simulink model "Parallel_Inverter_Functional1"  (R2021a)
settings: Solver=ode23tb  StartTime=0.0  StopTime=2  RelTol=1e-3
InitFcn:
  | fsw=10e3;
  | Ts=50e-6;
  | Vodref=400*sqrt(2/3);
  | Vdc= 700;
  | w0=2*pi*50;
  | Vdref=400*sqrt(2/3);
  | Lf=3.5e-3;
  | Rf=0.1;
  | Cf=50e-6;
  | Lc1=0.3e-3;
  | Rc1=0.01;
  | Lc2=0.8e-3;
  | Rc2=0.05;
  | 
  | 
  | Tci=4/(2*pi*fsw);
  | wci=1/Tci;
  | Kpc=Lf*wci;
  | Kic=Rf*wci;
  | 
  | pm=50;
  | wcv=1/Tci*(1-sind(pm))/(1+sind(pm));
  | wgc=sqrt(wcv*wci);
  | Kpv=Cf*wgc;
  | Kiv=Kpv*wcv;
  | PLoad = 3000*0.8;
  | QLoad = 3000*0.6;
  | 
  | m1=5e-5;
  | n1=3e-4;
  | m2=2e-5;
  | n2=1e-4;
libraries: spsThreePhaseSeriesRLCBranchLib x6, spsabctodq0Lib x6, spsThreePhaseVIMeasurementLib x5, spsDCVoltageSourceLib x2, spsPWMGenerator2LevelLib x2, spsUniversalBridgeLib x2, spsGroundLib x2, spsdq0toabcLib x2, spsThreePhaseSeriesRLCLoadLib x2, spsThreePhaseBreakerLib x1, spspowerguiLib x1
settings Model: SimulationMode=accelerator  Creator=adarshadhungel1  LastModifiedBy=Electrical
settings SolverCC: AlgebraicLoopSolver=TrustRegion
settings DataIOCC: LoggingToFile=on
settings DebuggingCC: SFMachineParentedDataDiag=warning  ArithmeticOperatorsInVariantConditions=warning
settings SFSimCC: SimUseLocalCustomCode=off  CustomCodeUndefinedFunction=UseInterfaceOnly
settings RTWCC: RTWUseLocalCustomCode=off

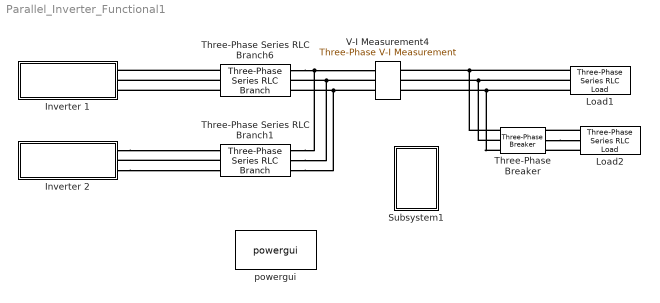
== system Parallel_Inverter_Functional1 ==
  Inverter 1 : Subsystem
  Inverter 2 : Subsystem
  Load1 : spsThreePhaseSeriesRLCLoadLib/Three-Phase Series RLC Load  LConnTagsString=A|B|C  Configuration=Y (grounded)  NominalVoltage=400  Vabc=[1e3 1e3 1e3]  Vabcp=[1e3 1e3 1e3]  NominalFrequency=50  UnbalancedPower=off  ActivePower=PLoad  InductivePower=QLoad  CapacitivePower=0  Pabc=[10e3 9e3 11e3]  QLabc=[100 90 110]  QCabc=[100 90 110]  Pabcp=[10e3 9e3 11e3]  QLabcp=[100 90 110]  QCabcp=[100 90 110]  Measurements=None  LoadType=constant Z
  Load2 : spsThreePhaseSeriesRLCLoadLib/Three-Phase Series RLC Load  LConnTagsString=A|B|C  Configuration=Y (grounded)  NominalVoltage=400  Vabc=[1e3 1e3 1e3]  Vabcp=[1e3 1e3 1e3]  NominalFrequency=50  UnbalancedPower=off  ActivePower=800  InductivePower=600  CapacitivePower=0  Pabc=[10e3 9e3 11e3]  QLabc=[100 90 110]  QCabc=[100 90 110]  Pabcp=[10e3 9e3 11e3]  QLabcp=[100 90 110]  QCabcp=[100 90 110]  Measurements=None  LoadType=constant Z
  Subsystem1 : Subsystem
  Three-Phase Series RLC Branch1 : spsThreePhaseSeriesRLCBranchLib/Three-Phase Series RLC Branch  LConnTagsString=A|B|C  RConnTagsString=A|B|C  BranchType=RL  Resistance=Rc2  Inductance=Lc2  Capacitance=1e-6  Measurements=None
  Three-Phase Series RLC Branch6 : spsThreePhaseSeriesRLCBranchLib/Three-Phase Series RLC Branch  LConnTagsString=A|B|C  RConnTagsString=A|B|C  BranchType=RL  Resistance=Rc1  Inductance=Lc1  Capacitance=1e-6  Measurements=None
  Three-Phase Breaker : spsThreePhaseBreakerLib/Three-Phase Breaker  InitialState=open  SwitchA=on  SwitchB=on  SwitchC=on  SwitchTimes="[1  2]"  External=off  BreakerResistance=0.01  SnubberResistance=1e6  SnubberCapacitance=inf  Measurements=None
  V-I Measurement4 : spsThreePhaseVIMeasurementLib/Three-Phase V-I Measurement  VoltageMeasurement=phase-to-ground  SetLabelV=on  LabelV=VLoad  Vpu=off  VpuLL=off  CurrentMeasurement=yes  SetLabelI=on  LabelI=ILoad  Ipu=off  Pbase=100e6  Vbase=500e3  OutputType=Complex  PhasorSimulation=off  PSBequivalent=0
  powergui : spspowerguiLib/powergui  Priority=1  SimulationMode=Discrete  SampleTime=Ts  frequency=60  Iterations=50  frequencyindice=0  Pbase=100e6  ErrMax=1e-4  UnitsV=kV  UnitsW=MW  buscounter=0  FunctionMessages=off  echomessages=off  EnableUseOfTLC=off  CurrentSourceSwitches=off  DisableSnubberDevices=off  DisableRonSwitches=off  DisableVfSwitches=off  DisplayEquations=off  AutomaticDiscreteSolvers=off  SolverType=Tustin/Backward Euler (TBE)  Interpol=off  ExternalGateDelay=off  methode=off  Ts=100  x0status=blocks  SPID=on  SwTol=0  HookPort=off  NonlinearTolerance=1e-4  nMaxIteration=100  ContinueOnMaxIteration=off  RestoreLinks=warning  ResistiveCurrentMeasurement=off  Frange=[0:2:500]  Ylog=off  Xlog=on  ShowGrid=off  save=off  variable=ZData  structure=VI1  ZoomFFT=off  StartTime=0  cycles=5  DisplayStyle=2  fundamental=50  FreqAxis=off  MaxFrequency=600  frequencyindicesteady=1  RmsSteady=1  display=off
  connections:
  Load1/LConn1 -- Three-Phase Breaker/LConn1 -- V-I Measurement4/RConn1
  Load1/LConn2 -- Three-Phase Breaker/LConn2 -- V-I Measurement4/RConn2
  Load1/LConn3 -- Three-Phase Breaker/LConn3 -- V-I Measurement4/RConn3
  Three-Phase Series RLC Branch6/RConn1 -- Three-Phase Series RLC Branch1/RConn1 -- V-I Measurement4/LConn1
  V-I Measurement4/LConn2 -- Three-Phase Series RLC Branch1/RConn2 -- Three-Phase Series RLC Branch6/RConn2
  V-I Measurement4/LConn3 -- Three-Phase Series RLC Branch1/RConn3 -- Three-Phase Series RLC Branch6/RConn3
  Three-Phase Series RLC Branch6/LConn1 -- Inverter 1/RConn1
  Three-Phase Series RLC Branch6/LConn2 -- Inverter 1/RConn2
  Three-Phase Series RLC Branch6/LConn3 -- Inverter 1/RConn3
  Inverter 2/RConn1 -- Three-Phase Series RLC Branch1/LConn1
  Three-Phase Series RLC Branch1/LConn2 -- Inverter 2/RConn2
  Inverter 2/RConn3 -- Three-Phase Series RLC Branch1/LConn3
  Load2/LConn1 -- Three-Phase Breaker/RConn1
  Three-Phase Breaker/RConn2 -- Load2/LConn2
  Load2/LConn3 -- Three-Phase Breaker/RConn3

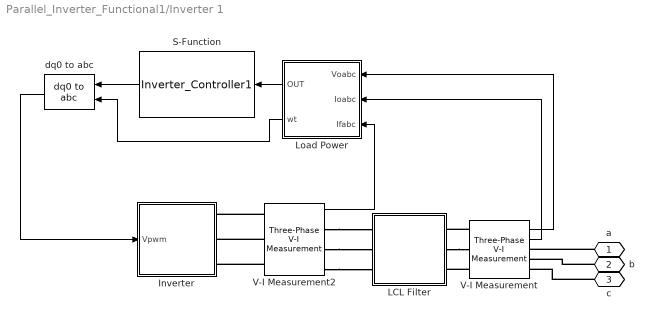
== system Parallel_Inverter_Functional1/Inverter 1 ==
  Inverter : Subsystem
  LCL Filter : Subsystem
  "Load Power " : Subsystem
  S-Function : S-Function  FunctionName=Inverter_Controller1  Parameters=Lf ,Cf  SFunctionDeploymentMode=off  EnableBusSupport=off
  V-I Measurement : spsThreePhaseVIMeasurementLib/Three-Phase V-I Measurement  VoltageMeasurement=phase-to-ground  SetLabelV=off  LabelV=Voabc  Vpu=off  VpuLL=off  CurrentMeasurement=yes  SetLabelI=off  LabelI=Ioabc  Ipu=off  Pbase=100e6  Vbase=500e3  OutputType=Complex  PhasorSimulation=off  PSBequivalent=0
  V-I Measurement2 : spsThreePhaseVIMeasurementLib/Three-Phase V-I Measurement  VoltageMeasurement=phase-to-ground  SetLabelV=on  LabelV=Viabc1  Vpu=off  VpuLL=off  CurrentMeasurement=yes  SetLabelI=off  LabelI=Ifabc  Ipu=off  Pbase=100e6  Vbase=500e3  OutputType=Complex  PhasorSimulation=off  PSBequivalent=0
  dq0 to abc : spsdq0toabcLib/dq0 to abc  Alignment=90 degrees behind phase A axis
  a : PMIOPort  Side=Right
  b : PMIOPort  Port=2  Side=Right
  c : PMIOPort  Port=3  Side=Right
  wires:
  "Load Power "/1(OUT) -> S-Function/1
  V-I Measurement/1 -> "Load Power "/1(Voabc)
  V-I Measurement/2 -> "Load Power "/2(Ioabc)
  V-I Measurement2/1 -> "Load Power "/3(Ifabc)
  S-Function/1 -> dq0 to abc/1
  "Load Power "/2(wt) -> dq0 to abc/2
  dq0 to abc/1 -> Inverter/1(Vpwm)
  connections:
  V-I Measurement2/LConn1 -- Inverter/RConn1
  V-I Measurement2/RConn1 -- LCL Filter/LConn1
  V-I Measurement/LConn3 -- LCL Filter/RConn3
  V-I Measurement2/LConn2 -- Inverter/RConn2
  V-I Measurement2/RConn2 -- LCL Filter/LConn2
  V-I Measurement2/LConn3 -- Inverter/RConn3
  V-I Measurement2/RConn3 -- LCL Filter/LConn3
  V-I Measurement/LConn1 -- LCL Filter/RConn1
  LCL Filter/RConn2 -- V-I Measurement/LConn2
  c/RConn1 -- V-I Measurement/RConn3
  b/RConn1 -- V-I Measurement/RConn2
  a/RConn1 -- V-I Measurement/RConn1

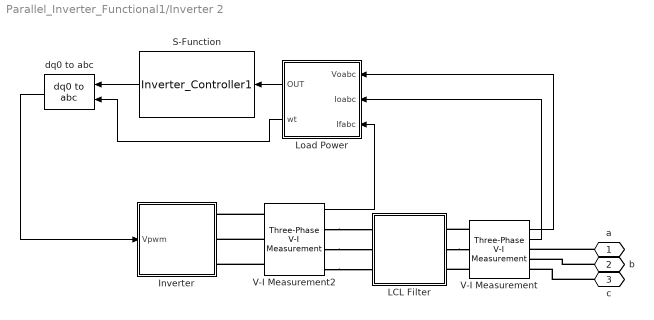
== system Parallel_Inverter_Functional1/Inverter 2 ==
  Inverter : Subsystem
  LCL Filter : Subsystem
  "Load Power " : Subsystem
  S-Function : S-Function  FunctionName=Inverter_Controller1  Parameters=Lf,Cf  SFunctionDeploymentMode=off  EnableBusSupport=off
  V-I Measurement : spsThreePhaseVIMeasurementLib/Three-Phase V-I Measurement  VoltageMeasurement=phase-to-ground  SetLabelV=off  LabelV=Voabc  Vpu=off  VpuLL=off  CurrentMeasurement=yes  SetLabelI=off  LabelI=Ioabc  Ipu=off  Pbase=100e6  Vbase=500e3  OutputType=Complex  PhasorSimulation=off  PSBequivalent=0
  V-I Measurement2 : spsThreePhaseVIMeasurementLib/Three-Phase V-I Measurement  VoltageMeasurement=phase-to-ground  SetLabelV=on  LabelV=Viabc  Vpu=off  VpuLL=off  CurrentMeasurement=yes  SetLabelI=off  LabelI=Ifabc  Ipu=off  Pbase=100e6  Vbase=500e3  OutputType=Complex  PhasorSimulation=off  PSBequivalent=0
  dq0 to abc : spsdq0toabcLib/dq0 to abc  Alignment=90 degrees behind phase A axis
  a : PMIOPort  Side=Right
  b : PMIOPort  Port=2  Side=Right
  c : PMIOPort  Port=3  Side=Right
  wires:
  dq0 to abc/1 -> Inverter/1(Vpwm)
  "Load Power "/2(wt) -> dq0 to abc/2
  S-Function/1 -> dq0 to abc/1
  V-I Measurement2/1 -> "Load Power "/3(Ifabc)
  V-I Measurement/2 -> "Load Power "/2(Ioabc)
  V-I Measurement/1 -> "Load Power "/1(Voabc)
  "Load Power "/1(OUT) -> S-Function/1
  connections:
  a/RConn1 -- V-I Measurement/RConn1
  b/RConn1 -- V-I Measurement/RConn2
  c/RConn1 -- V-I Measurement/RConn3
  LCL Filter/RConn2 -- V-I Measurement/LConn2
  V-I Measurement/LConn1 -- LCL Filter/RConn1
  V-I Measurement2/RConn3 -- LCL Filter/LConn3
  V-I Measurement2/LConn3 -- Inverter/RConn3
  V-I Measurement2/RConn2 -- LCL Filter/LConn2
  V-I Measurement2/LConn2 -- Inverter/RConn2
  V-I Measurement/LConn3 -- LCL Filter/RConn3
  V-I Measurement2/RConn1 -- LCL Filter/LConn1
  V-I Measurement2/LConn1 -- Inverter/RConn1

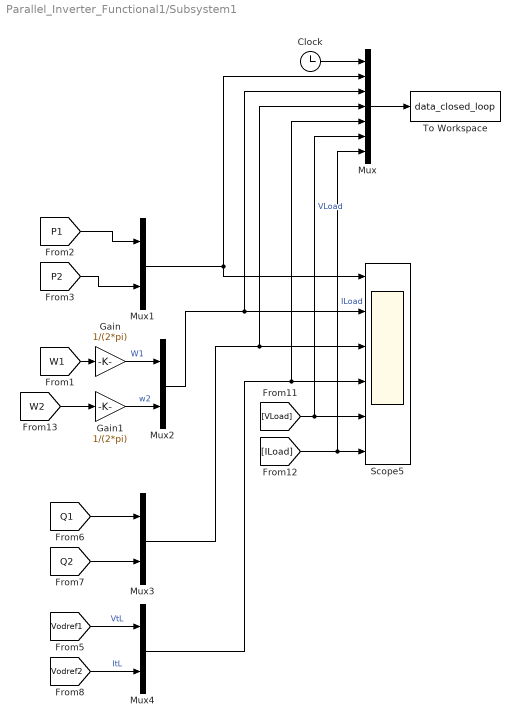
== system Parallel_Inverter_Functional1/Subsystem1 ==
  Clock : Clock
  Gain : Gain  Gain=1/(2*pi)
  Gain1 : Gain  Gain=1/(2*pi)
  Mux : Mux  Inputs=7
  Mux{1..4} (4 alike) : Mux  Inputs=2
  Scope5 : Scope  NumInputPorts=6
  To Workspace : ToWorkspace  VariableName=data_closed_loop  SampleTime=0.001
  wires:
  Mux3/1 -> Mux/4, Scope5/3
  Mux1/1 -> Scope5/1, Mux/2
  [Q1] -> Mux3/1
  [P1] -> Mux1/1
  Gain/1 -> Mux2/1  "W1"
  Mux4/1 -> Mux/5, Scope5/4
  [W2] -> Gain1/1
  [Vodref2] -> Mux4/2  "ItL"
  Mux2/1 -> Mux/3, Scope5/2
  Gain1/1 -> Mux2/2  "w2"
  [Q2] -> Mux3/2
  [VLoad] -> Mux/6, Scope5/5  "VLoad"
  [ILoad] -> Mux/7, Scope5/6  "ILoad"
  Clock/1 -> Mux/1
  [P2] -> Mux1/2
  Mux/1 -> To Workspace/1
  [W1] -> Gain/1
  [Vodref1] -> Mux4/1  "VtL"

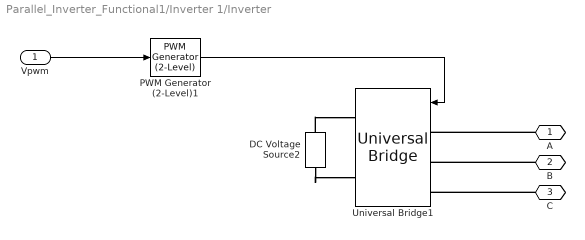
== system Parallel_Inverter_Functional1/Inverter 1/Inverter ==
  Vpwm : Inport
  DC Voltage Source2 : spsDCVoltageSourceLib/DC Voltage Source  Amplitude=Vdc  Measurements=None
  PWM Generator (2-Level)1 : spsPWMGenerator2LevelLib/PWM Generator (2-Level)  ModulatorType=Three-phase bridge (6 pulses)  ModulatorMode=Unsynchronized  Fc=fsw  Pc=0  nF=27  MinMax="[ -1  1 ]"  SamplingTechnique=Natural  ModulatingSignals=off  m=0.8  Freq=60  Phase=0  Ts=0  ShowCarrierOutport=off
  Universal Bridge1 : spsUniversalBridgeLib/Universal Bridge  Arms=3  SnubberResistance=1e5  SnubberCapacitance=inf  Device=IGBT / Diodes  Ron=1e-3  Lon=0  ForwardVoltages="[  0  0  ]"  ForwardVoltage=0  GTOparameters=[ 10e-6 , 20e-6 ]  IGBTparameters=[ 1e-6 , 2e-6 ]  Measurements=None  Measurements_2=None  converterType=Rectifier
  A : PMIOPort  Side=Right
  B : PMIOPort  Port=2  Side=Right
  C : PMIOPort  Port=3  Side=Right
  wires:
  PWM Generator (2-Level)1/1 -> Universal Bridge1/1
  Vpwm/1 -> PWM Generator (2-Level)1/1
  connections:
  A/RConn1 -- Universal Bridge1/LConn1
  C/RConn1 -- Universal Bridge1/LConn3
  DC Voltage Source2/LConn1 -- Universal Bridge1/RConn2
  DC Voltage Source2/RConn1 -- Universal Bridge1/RConn1
  B/RConn1 -- Universal Bridge1/LConn2

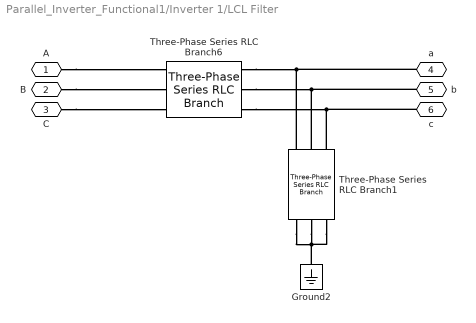
== system Parallel_Inverter_Functional1/Inverter 1/LCL Filter ==
  Ground2 : spsGroundLib/Ground  LConnTagsString=a
  Three-Phase Series RLC Branch1 : spsThreePhaseSeriesRLCBranchLib/Three-Phase Series RLC Branch  LConnTagsString=A|B|C  RConnTagsString=A|B|C  BranchType=C  Resistance=0.15  Inductance=3.5e-4  Capacitance=Cf  Measurements=None
  Three-Phase Series RLC Branch6 : spsThreePhaseSeriesRLCBranchLib/Three-Phase Series RLC Branch  LConnTagsString=A|B|C  RConnTagsString=A|B|C  BranchType=RL  Resistance=Rf  Inductance=Lf  Capacitance=1e-6  Measurements=None
  A : PMIOPort  Side=Left
  B : PMIOPort  Port=2  Side=Left
  C : PMIOPort  Port=3  Side=Left
  a : PMIOPort  Port=4  Side=Right
  b : PMIOPort  Port=5  Side=Right
  c : PMIOPort  Port=6  Side=Right
  connections:
  Three-Phase Series RLC Branch1/LConn1 -- a/RConn1 -- Three-Phase Series RLC Branch6/RConn1
  Three-Phase Series RLC Branch1/LConn3 -- c/RConn1 -- Three-Phase Series RLC Branch6/RConn3
  Three-Phase Series RLC Branch1/LConn2 -- Three-Phase Series RLC Branch6/RConn2 -- b/RConn1
  Three-Phase Series RLC Branch1/RConn3 -- Three-Phase Series RLC Branch1/RConn1 -- Ground2/LConn1 -- Three-Phase Series RLC Branch1/RConn2
  A/RConn1 -- Three-Phase Series RLC Branch6/LConn1
  B/RConn1 -- Three-Phase Series RLC Branch6/LConn2
  C/RConn1 -- Three-Phase Series RLC Branch6/LConn3

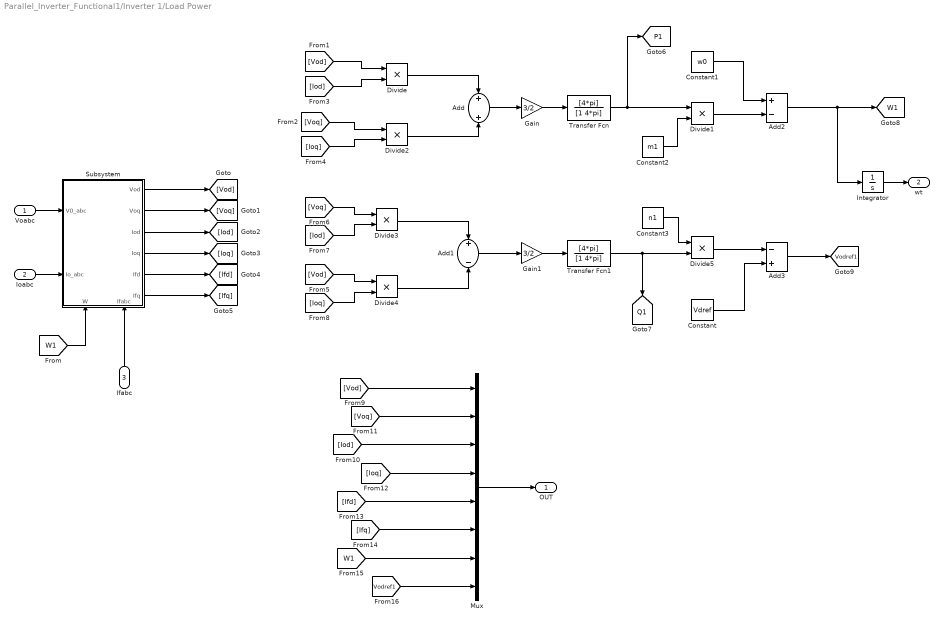
== system Parallel_Inverter_Functional1/Inverter 1/Load Power  ==
  Voabc : Inport
  Ioabc : Inport  Port=2
  Ifabc : Inport  Port=3
  Add : Sum
  Add1 : Sum  Inputs=+-
  Add2 : Sum  Inputs=+-
  Add3 : Sum  Inputs=-+
  Constant : Constant  Value=Vdref
  Constant1 : Constant  Value=w0
  Constant2 : Constant  Value=m1
  Constant3 : Constant  Value=n1
  Divide{,1..5} (6 alike) : Product  Inputs=**
  Gain : Gain  Gain=3/2
  Gain1 : Gain  Gain=3/2
  Integrator : Integrator
  Mux : Mux  Inputs=8
  Subsystem : Subsystem
      settings: PortSchema="{\"entries\":[{\"content\":{\"sides\":[{\"content\":{\"connectorIds\":[\"In1\",\"In2\"]},\"type\":\"ConnectorPlacement.EquallySpacedRectSide\",\"uuid\":\"3c0ce44c-1409-4df9-aab1-2e1a82b43481\"},{\"content\":{\"connectorIds\":[\"Out1\",\"Out2\",\"Out3\",\"Out4\",\"Out5\",\"Out6\"],\"side\":\"RIGHT\"},\"type\":\"ConnectorPlacement.EquallySpacedRectSide\",\"uuid\":\"4a9336a4-679f-4f93-987c-a9f8549bd21c\"},{\"content\":{\"connectorIds\":[],\"side\":\"TOP\"},\"type\":\"ConnectorPlacement.EquallySpacedRectSide\",\"uuid\":\"6340f487-ff74-466e-845e-7d1050881641\"},{\"content\":{\"connectorIds\":[\"In3\",\"In4\"],\"side\":\"BOTTOM\"},\"type\":\"ConnectorPlacement.EquallySpacedRectSide\",\"uuid\":\"1e1d92d0-8955-434a-9fbd-76af504505ea\"}]},\"type\":\"ConnectorPlacement.EquallySpacedConnector\",\"uuid\":\"bfddd833-a64a-4f18-a4bd-88042aac52a3\"}],\"packageUris\":[\"http://schema.mathworks.com/mf0/Connector/R2020b\"],\"version\":\"1.0\"}"
  Transfer Fcn : TransferFcn  Numerator=[4*pi]  Denominator=[1 4*pi]  ParameterTunability=Optimized
  Transfer Fcn1 : TransferFcn  Numerator=[4*pi]  Denominator=[1 4*pi]  ParameterTunability=Optimized
  OUT : Outport
  wt : Outport  Port=2
  tag scope: P1=global, Q1=global, Vodref1=global, W1=global
  wires:
  Voabc/1 -> Subsystem/1(V0_abc)
  Gain/1 -> Transfer Fcn/1
  Constant3/1 -> Divide5/1
  Ioabc/1 -> Subsystem/2(Io_abc)
  Subsystem/2(Voq) -> [Voq]
  Transfer Fcn1/1 -> [Q1], Divide5/2
  Gain1/1 -> Transfer Fcn1/1
  Add2/1 -> Integrator/1, [W1]
  Transfer Fcn/1 -> [P1], Divide1/1
  Subsystem/3(Iod) -> [Iod]
  Add3/1 -> [Vodref1]
  Divide5/1 -> Add3/1
  Divide/1 -> Add/1
  Divide1/1 -> Add2/2
  Add1/1 -> Gain1/1
  Add/1 -> Gain/1
  Constant2/1 -> Divide1/2
  Divide3/1 -> Add1/1
  Constant1/1 -> Add2/1
  [Ioq] -> Divide2/2
  [Vod] -> Divide4/1
  [Ioq] -> Divide4/2
  Constant/1 -> Add3/2
  Divide2/1 -> Add/2
  [Iod] -> Divide3/2
  Divide4/1 -> Add1/2
  [Voq] -> Divide3/1
  Subsystem/4(Ioq) -> [Ioq]
  [Voq] -> Divide2/1
  Subsystem/1(Vod) -> [Vod]
  [Vod] -> Divide/1
  [Iod] -> Divide/2
  Subsystem/5(Ifd) -> [Ifd]
  Subsystem/6(Ifq) -> [Ifq]
  Ifabc/1 -> Subsystem/4(Ifabc)
  [Vod] -> Mux/1
  [Iod] -> Mux/3
  [Ioq] -> Mux/4
  [Voq] -> Mux/2
  [Ifd] -> Mux/5
  [Ifq] -> Mux/6
  [W1] -> Mux/7
  [Vodref1] -> Mux/8
  Mux/1 -> OUT/1
  Integrator/1 -> wt/1
  [W1] -> Subsystem/3(W)

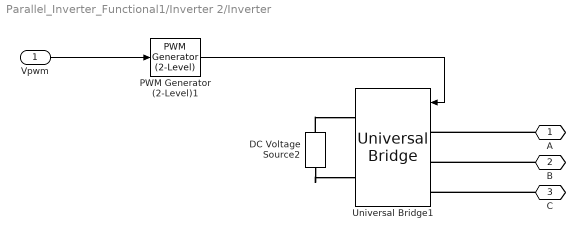
== system Parallel_Inverter_Functional1/Inverter 2/Inverter ==
  Vpwm : Inport
  DC Voltage Source2 : spsDCVoltageSourceLib/DC Voltage Source  Amplitude=Vdc  Measurements=None
  PWM Generator (2-Level)1 : spsPWMGenerator2LevelLib/PWM Generator (2-Level)  ModulatorType=Three-phase bridge (6 pulses)  ModulatorMode=Unsynchronized  Fc=fsw  Pc=0  nF=27  MinMax="[ -1  1 ]"  SamplingTechnique=Natural  ModulatingSignals=off  m=0.8  Freq=60  Phase=0  Ts=0  ShowCarrierOutport=off
  Universal Bridge1 : spsUniversalBridgeLib/Universal Bridge  Arms=3  SnubberResistance=1e5  SnubberCapacitance=inf  Device=IGBT / Diodes  Ron=1e-3  Lon=0  ForwardVoltages="[  0  0  ]"  ForwardVoltage=0  GTOparameters=[ 10e-6 , 20e-6 ]  IGBTparameters=[ 1e-6 , 2e-6 ]  Measurements=None  Measurements_2=None  converterType=Rectifier
  A : PMIOPort  Side=Right
  B : PMIOPort  Port=2  Side=Right
  C : PMIOPort  Port=3  Side=Right
  wires:
  Vpwm/1 -> PWM Generator (2-Level)1/1
  PWM Generator (2-Level)1/1 -> Universal Bridge1/1
  connections:
  B/RConn1 -- Universal Bridge1/LConn2
  DC Voltage Source2/RConn1 -- Universal Bridge1/RConn1
  DC Voltage Source2/LConn1 -- Universal Bridge1/RConn2
  C/RConn1 -- Universal Bridge1/LConn3
  A/RConn1 -- Universal Bridge1/LConn1

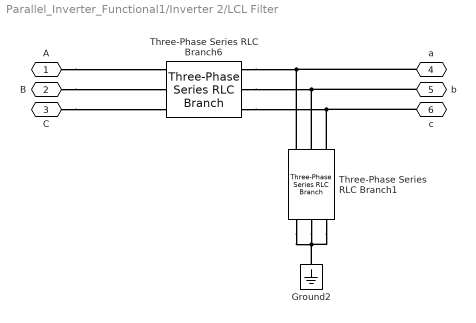
== system Parallel_Inverter_Functional1/Inverter 2/LCL Filter ==
  Ground2 : spsGroundLib/Ground  LConnTagsString=a
  Three-Phase Series RLC Branch1 : spsThreePhaseSeriesRLCBranchLib/Three-Phase Series RLC Branch  LConnTagsString=A|B|C  RConnTagsString=A|B|C  BranchType=C  Resistance=0.15  Inductance=3.5e-4  Capacitance=Cf  Measurements=None
  Three-Phase Series RLC Branch6 : spsThreePhaseSeriesRLCBranchLib/Three-Phase Series RLC Branch  LConnTagsString=A|B|C  RConnTagsString=A|B|C  BranchType=RL  Resistance=Rf  Inductance=Lf  Capacitance=1e-6  Measurements=None
  A : PMIOPort  Side=Left
  B : PMIOPort  Port=2  Side=Left
  C : PMIOPort  Port=3  Side=Left
  a : PMIOPort  Port=4  Side=Right
  b : PMIOPort  Port=5  Side=Right
  c : PMIOPort  Port=6  Side=Right
  connections:
  C/RConn1 -- Three-Phase Series RLC Branch6/LConn3
  B/RConn1 -- Three-Phase Series RLC Branch6/LConn2
  A/RConn1 -- Three-Phase Series RLC Branch6/LConn1
  Three-Phase Series RLC Branch1/RConn2 -- Ground2/LConn1 -- Three-Phase Series RLC Branch1/RConn1 -- Three-Phase Series RLC Branch1/RConn3
  b/RConn1 -- Three-Phase Series RLC Branch6/RConn2 -- Three-Phase Series RLC Branch1/LConn2
  Three-Phase Series RLC Branch6/RConn3 -- c/RConn1 -- Three-Phase Series RLC Branch1/LConn3
  Three-Phase Series RLC Branch6/RConn1 -- a/RConn1 -- Three-Phase Series RLC Branch1/LConn1

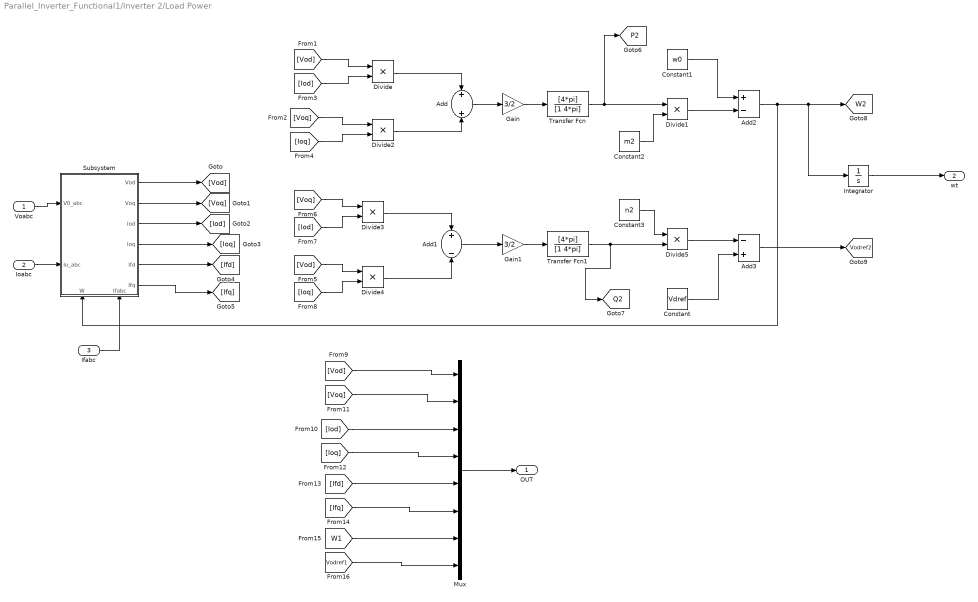
== system Parallel_Inverter_Functional1/Inverter 2/Load Power  ==
  Voabc : Inport
  Ioabc : Inport  Port=2
  Ifabc : Inport  Port=3
  Add : Sum
  Add1 : Sum  Inputs=+-
  Add2 : Sum  Inputs=+-
  Add3 : Sum  Inputs=-+
  Constant : Constant  Value=Vdref
  Constant1 : Constant  Value=w0
  Constant2 : Constant  Value=m2
  Constant3 : Constant  Value=n2
  Divide{,1..5} (6 alike) : Product  Inputs=**
  Gain : Gain  Gain=3/2
  Gain1 : Gain  Gain=3/2
  Integrator : Integrator
  Mux : Mux  Inputs=8
  Subsystem : Subsystem
      settings: PortSchema="{\"entries\":[{\"content\":{\"sides\":[{\"content\":{\"connectorIds\":[\"In1\",\"In2\"]},\"type\":\"ConnectorPlacement.EquallySpacedRectSide\",\"uuid\":\"3c0ce44c-1409-4df9-aab1-2e1a82b43481\"},{\"content\":{\"connectorIds\":[\"Out1\",\"Out2\",\"Out3\",\"Out4\",\"Out5\",\"Out6\"],\"side\":\"RIGHT\"},\"type\":\"ConnectorPlacement.EquallySpacedRectSide\",\"uuid\":\"4a9336a4-679f-4f93-987c-a9f8549bd21c\"},{\"content\":{\"connectorIds\":[],\"side\":\"TOP\"},\"type\":\"ConnectorPlacement.EquallySpacedRectSide\",\"uuid\":\"6340f487-ff74-466e-845e-7d1050881641\"},{\"content\":{\"connectorIds\":[\"In3\",\"In4\"],\"side\":\"BOTTOM\"},\"type\":\"ConnectorPlacement.EquallySpacedRectSide\",\"uuid\":\"1e1d92d0-8955-434a-9fbd-76af504505ea\"}]},\"type\":\"ConnectorPlacement.EquallySpacedConnector\",\"uuid\":\"bfddd833-a64a-4f18-a4bd-88042aac52a3\"}],\"packageUris\":[\"http://schema.mathworks.com/mf0/Connector/R2020b\"],\"version\":\"1.0\"}"
  Transfer Fcn : TransferFcn  Numerator=[4*pi]  Denominator=[1 4*pi]  ParameterTunability=Optimized
  Transfer Fcn1 : TransferFcn  Numerator=[4*pi]  Denominator=[1 4*pi]  ParameterTunability=Optimized
  OUT : Outport
  wt : Outport  Port=2
  tag scope: P2=global, Q2=global, Vodref2=global, W2=global
  wires:
  Integrator/1 -> wt/1
  Mux/1 -> OUT/1
  [Vodref1] -> Mux/8
  [W1] -> Mux/7
  [Ifq] -> Mux/6
  [Ifd] -> Mux/5
  [Voq] -> Mux/2
  [Ioq] -> Mux/4
  [Iod] -> Mux/3
  [Vod] -> Mux/1
  Ifabc/1 -> Subsystem/4(Ifabc)
  Subsystem/6(Ifq) -> [Ifq]
  Subsystem/5(Ifd) -> [Ifd]
  [Iod] -> Divide/2
  [Vod] -> Divide/1
  Subsystem/1(Vod) -> [Vod]
  [Voq] -> Divide2/1
  Subsystem/4(Ioq) -> [Ioq]
  [Voq] -> Divide3/1
  Divide4/1 -> Add1/2
  [Iod] -> Divide3/2
  Divide2/1 -> Add/2
  Constant/1 -> Add3/2
  [Ioq] -> Divide4/2
  [Vod] -> Divide4/1
  [Ioq] -> Divide2/2
  Constant1/1 -> Add2/1
  Divide3/1 -> Add1/1
  Constant2/1 -> Divide1/2
  Add/1 -> Gain/1
  Add1/1 -> Gain1/1
  Divide1/1 -> Add2/2
  Divide/1 -> Add/1
  Divide5/1 -> Add3/1
  Add3/1 -> [Vodref2]
  Subsystem/3(Iod) -> [Iod]
  Transfer Fcn/1 -> Divide1/1, [P2]
  Add2/1 -> Subsystem/3(W), [W2], Integrator/1
  Gain1/1 -> Transfer Fcn1/1
  Transfer Fcn1/1 -> Divide5/2, [Q2]
  Subsystem/2(Voq) -> [Voq]
  Ioabc/1 -> Subsystem/2(Io_abc)
  Constant3/1 -> Divide5/1
  Gain/1 -> Transfer Fcn/1
  Voabc/1 -> Subsystem/1(V0_abc)

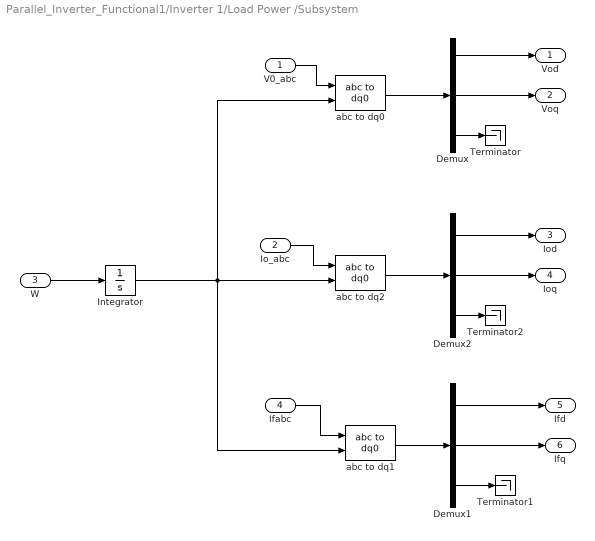
== system Parallel_Inverter_Functional1/Inverter 1/Load Power /Subsystem ==
  V0_abc : Inport
  Io_abc : Inport  Port=2
  W : Inport  Port=3
  Ifabc : Inport  Port=4
  Demux : Demux  Outputs=3
  Demux1 : Demux  Outputs=3
  Demux2 : Demux  Outputs=3
  Integrator : Integrator
  Terminator : Terminator
  Terminator1 : Terminator
  Terminator2 : Terminator
  abc to dq0 : spsabctodq0Lib/abc to dq0  Alignment=90 degrees behind phase A axis
  abc to dq1 : spsabctodq0Lib/abc to dq0  Alignment=90 degrees behind phase A axis
  abc to dq2 : spsabctodq0Lib/abc to dq0  Alignment=90 degrees behind phase A axis
  Vod : Outport
  Voq : Outport  Port=2
  Iod : Outport  Port=3
  Ioq : Outport  Port=4
  Ifd : Outport  Port=5
  Ifq : Outport  Port=6
  wires:
  abc to dq2/1 -> Demux2/1
  Demux/2 -> Voq/1
  Integrator/1 -> abc to dq0/2, abc to dq1/2, abc to dq2/2
  Demux2/2 -> Ioq/1
  abc to dq0/1 -> Demux/1
  Demux2/3 -> Terminator2/1
  Demux2/1 -> Iod/1
  Demux/1 -> Vod/1
  Demux/3 -> Terminator/1
  W/1 -> Integrator/1
  Io_abc/1 -> abc to dq2/1
  V0_abc/1 -> abc to dq0/1
  Ifabc/1 -> abc to dq1/1
  abc to dq1/1 -> Demux1/1
  Demux1/1 -> Ifd/1
  Demux1/2 -> Ifq/1
  Demux1/3 -> Terminator1/1

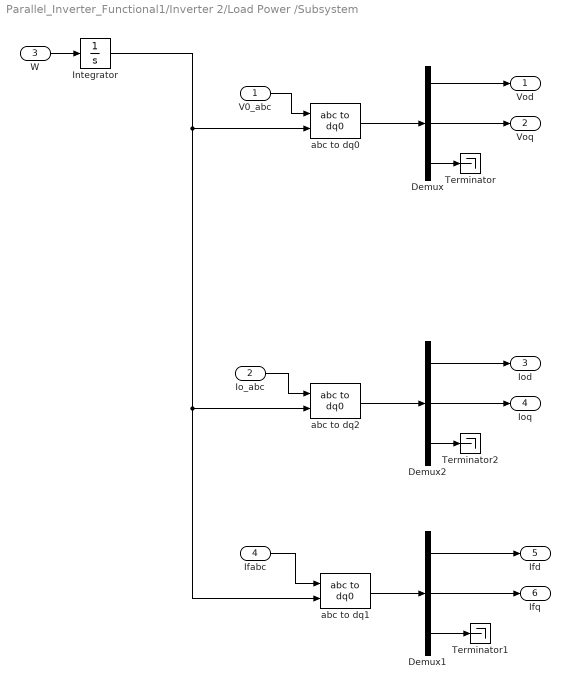
== system Parallel_Inverter_Functional1/Inverter 2/Load Power /Subsystem ==
  V0_abc : Inport
  Io_abc : Inport  Port=2
  W : Inport  Port=3
  Ifabc : Inport  Port=4
  Demux : Demux  Outputs=3
  Demux1 : Demux  Outputs=3
  Demux2 : Demux  Outputs=3
  Integrator : Integrator
  Terminator : Terminator
  Terminator1 : Terminator
  Terminator2 : Terminator
  abc to dq0 : spsabctodq0Lib/abc to dq0  Alignment=90 degrees behind phase A axis
  abc to dq1 : spsabctodq0Lib/abc to dq0  Alignment=90 degrees behind phase A axis
  abc to dq2 : spsabctodq0Lib/abc to dq0  Alignment=90 degrees behind phase A axis
  Vod : Outport
  Voq : Outport  Port=2
  Iod : Outport  Port=3
  Ioq : Outport  Port=4
  Ifd : Outport  Port=5
  Ifq : Outport  Port=6
  wires:
  Demux1/3 -> Terminator1/1
  Demux1/2 -> Ifq/1
  Demux1/1 -> Ifd/1
  abc to dq1/1 -> Demux1/1
  Ifabc/1 -> abc to dq1/1
  V0_abc/1 -> abc to dq0/1
  Io_abc/1 -> abc to dq2/1
  W/1 -> Integrator/1
  Demux/3 -> Terminator/1
  Demux/1 -> Vod/1
  Demux2/1 -> Iod/1
  Demux2/3 -> Terminator2/1
  abc to dq0/1 -> Demux/1
  Demux2/2 -> Ioq/1
  Integrator/1 -> abc to dq0/2, abc to dq2/2, abc to dq1/2
  Demux/2 -> Voq/1
  abc to dq2/1 -> Demux2/1
